simulink model "Constant_verif"  (Simulink 7.2)
settings: Solver=ode45  StartTime=0.0  StopTime=10.0  RelTol=1e-3
settings Model: Creator=Romain  LastModifiedBy=Romain
settings OptimizationCC: ExpressionDepthLimit=128
settings DebuggingCC: SolverPrmCheckMsg=none  FcnCallInpInsideContextMsg=Enable All  StateNameClashWarn=none  StrictBusMsg=ErrorLevel1
settings CodeAppCC: CustomSymbolStrType=$N$R$M_T
settings GRTTargetCC: TargetFunctionLibrary=C89/C90 (ANSI)

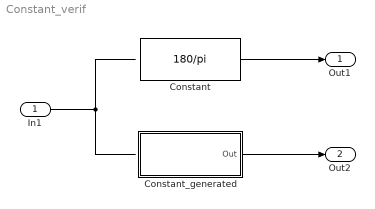
== system Constant_verif ==
  In1 : Inport  OutDataTypeStr=double  DataType=double
  Constant : Constant  Value=180/pi
  Constant_generated : Subsystem  TreatAsAtomicUnit=on
  Out1 : Outport
  Out2 : Outport  Port=2
  wires:
  In1/1 -> ?
  Constant/1 -> Out1/1
  Constant_generated/1(Out) -> Out2/1

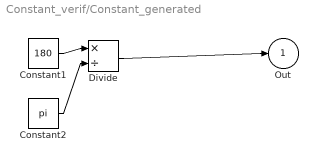
== system Constant_verif/Constant_generated ==
  Constant1 : Constant  Value=180
  Constant2 : Constant  Value=pi
  Divide : Product  Inputs=*/  SaturateOnIntegerOverflow=on  RndMeth=Zero  InputSameDT=on  OutDataTypeStr=Inherit: Same as first input
  Out : Outport
  wires:
  Divide/1 -> Out/1
  Constant1/1 -> Divide/1
  Constant2/1 -> Divide/2
